simulink model "Time_Varying_Model_2022b"  (R2023b)
settings: Solver=FixedStepAuto  StartTime=0.0  StopTime=10.899  FixedStep=0.01  RelTol=1e-3
values from neighbouring files (symbols this model uses):
  aptos = aptos.calcAeroCoeff(velocity)    [lqr_tuning_analysis.m]    (also in motor_speed_analysis.m; parameter_uncertainty.m; simulator.m; simulator_HIL.m)
  controller = controller.addGain(aptos, steadyState, velocity)    [lqr_tuning_analysis.m]    (also in motor_speed_analysis.m; parameter_uncertainty.m; robustness_analysis.m = controller.addGain(nominal, steadyState, velocity); simulator.m)
  OR = OpenRocketData('openrocket_data/OpenRocket_data_31-03-23.csv')    [robustness_analysis.m]
  q = 0.5 * obj.rho * obj.v^2    [Rocket.m]
  r = aptos    [parameter_uncertainty.m]
undefined symbols (not defined in the file or in its folder): F, Light, MIL
libraries: simulink_extras x20, aerolibutil x1, sharedtransform x1, simulink x1, aerolibwind2 x1
settings Model: Creator=mn19ty  LastModifiedBy=sambr
settings DataIOCC: ReturnWorkspaceOutputsName=yout
settings OptimizationCC: ReuseModelBlockBuffer=off
settings ModelReferenceCC: EnableRefExpFcnMdlSchedulingChecks=on

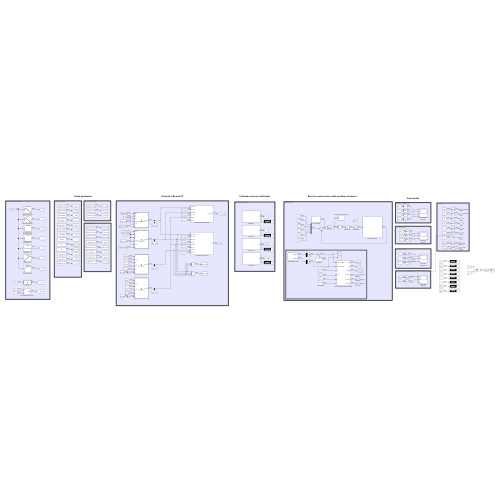
[thumbnail: Simulink's stored preview of the top-level diagram]
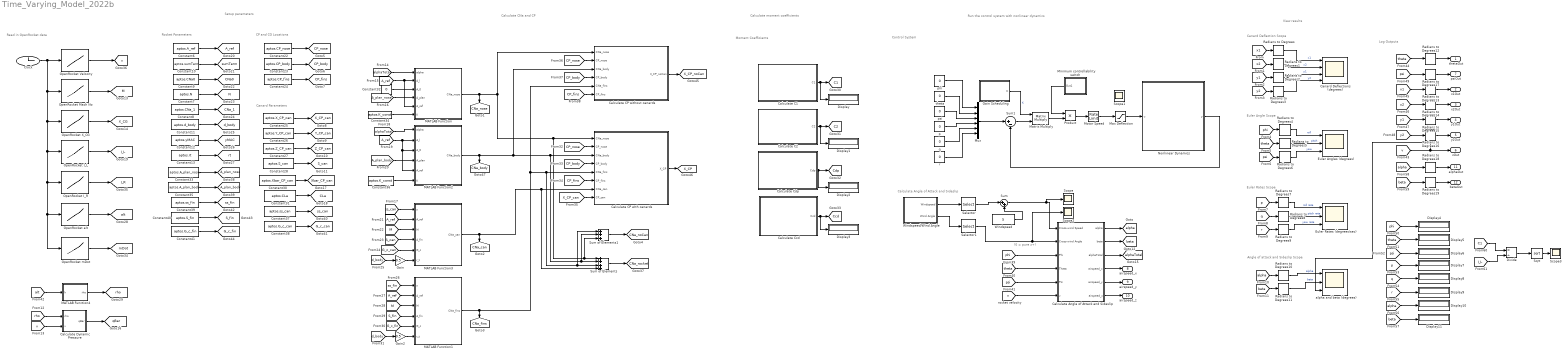
== system Time_Varying_Model_2022b ==
  note: (0 = pure z+)
  note: Log Outputs
  note: Read in OpenRocket data
  note: Calculate Angle of Attack and Sideslip
  note: Angle of attack and Sideslip Scope
  note: View results
  note: Run the control system with nonlinear dynamics
  note: Calculate moment coefficients
  note: Setup parameters
  note: Euler Rates Scope
  note: Euler Angle Scope
  note: Canard Deflection Scope
  note: Control System
  note: Moment Coefficients
  note: Rocket Parameters
  note: Canard Parameters
  note: CP and CG Locations
  note: Calculate CNa and CP
  Calculate Angle of Attack and Sideslip : Subsystem
  Calculate C1 : Subsystem
  Calculate C2 : Subsystem
  Calculate CP with canards : Subsystem
  Calculate CP without canards : Subsystem
  Calculate Ccd : Subsystem
  Calculate Cdp : Subsystem
  Calculate Dynamic Pressure : Subsystem
  Canard Deflections (degrees) : Scope  NumInputPorts=4
  Clock : Clock
  Constant10 : Constant  Value=aptos.sumTerm
  Constant11 : Constant  Value=aptos.d_body
  Constant12 : Constant  Value=aptos.yMAC
  Constant13 : Constant  Value=aptos.rt
  Constant22 : Constant  Value=aptos.CP_nose
  Constant23 : Constant  Value=aptos.CP_body
  Constant24 : Constant  Value=aptos.CP_fins
  Constant25 : Constant  Value=aptos.X_CP_can
  Constant26 : Constant  Value=aptos.Y_CP_can
  Constant27 : Constant  Value=aptos.Z_CP_can
  Constant28 : Constant  Value=aptos.S_can
  Constant30 : Constant  Value=aptos.Xbar_CP_can
  Constant31 : Constant  Value=aptos.CLa
  Constant32 : Constant  Value=0
  Constant33 : Constant  Value=aptos.A_plan_nose
  Constant34 : Constant  Value=aptos.K_const
  Constant35 : Constant  Value=aptos.A_plan_body
  Constant36 : Constant  Value=aptos.K_const
  Constant37 : Constant  Value=aptos.ss_can
  Constant38 : Constant  Value=aptos.G_c_can
  Constant39 : Constant  Value=aptos.ss_fin
  Constant40 : Constant  Value=aptos.S_fin
  Constant41 : Constant  Value=aptos.G_c_fin
  Constant6 : Constant  Value=aptos.A_ref
  Constant7 : Constant  Value=aptos.N
  Constant8 : Constant  Value=aptos.CNa_1
  Constant9 : Constant  Value=aptos.CNa0
  Display{,1..11} (12 alike) : Display
  Divide : Product  Inputs=*/
  Euler Angles (degrees) : Scope  NumInputPorts=3
  Euler Rates (degrees/sec) : Scope  NumInputPorts=3
  Gain : Gain  Gain=0.5
  Gain Scheduling : Subsystem
  Gain2 : Gain  Gain=0.5
  MATLAB Function : MATLAB Function  TreatAsAtomicUnit=on
  MATLAB Function1 : MATLAB Function  TreatAsAtomicUnit=on
  MATLAB Function2 : MATLAB Function  TreatAsAtomicUnit=on
  MATLAB Function3 : MATLAB Function  TreatAsAtomicUnit=on
  MATLAB Function4 : MATLAB Function  TreatAsAtomicUnit=on
  Matrix Multiply : Product  Multiplication=Matrix(*)
  Max Deflection : Saturate  UpperLimit=deg2rad(13)  LowerLimit=-deg2rad(13)
  Minimum controllability switch : Subsystem
  Motor Speed : RateLimiter  RisingSlewLimit=6.54  FallingSlewLimit=-6.54  SampleTimeMode=inherited
  Mux : Mux  Inputs=6
  Nonlinear Dynamics : Subsystem
  OpenRocket I_L : Lookup_n-D  NumberOfTableDimensions=1  BreakpointsForDimension1=OR.t  Table=OR.I_L  InternalRulePriority=Speed  RndMeth=Simplest
  OpenRocket I_R : Lookup_n-D  NumberOfTableDimensions=1  BreakpointsForDimension1=OR.t  Table=OR.I_R  InternalRulePriority=Speed  RndMeth=Simplest
  OpenRocket Mach No : Lookup_n-D  NumberOfTableDimensions=1  BreakpointsForDimension1=OR.t  Table=OR.M  InternalRulePriority=Speed  RndMeth=Simplest
  OpenRocket Velocity : Lookup_n-D  NumberOfTableDimensions=1  BreakpointsForDimension1=OR.t  Table=OR.v  InternalRulePriority=Speed  RndMeth=Simplest
  OpenRocket X_CG : Lookup_n-D  NumberOfTableDimensions=1  BreakpointsForDimension1=OR.t  Table=OR.X_CG  InternalRulePriority=Speed  RndMeth=Simplest
  OpenRocket alt : Lookup_n-D  NumberOfTableDimensions=1  BreakpointsForDimension1=OR.t  Table=OR.h  InternalRulePriority=Speed  RndMeth=Simplest
  OpenRocket mDot : Lookup_n-D  NumberOfTableDimensions=1  BreakpointsForDimension1=OR.t  Table=OR.mDot  InternalRulePriority=Speed  RndMeth=Simplest
  Product : Product
  Radians to Degrees{,1..19} (20 alike) : simulink_extras/Transformations/Radians to Degrees
  Scope{,1..3} (4 alike) : Scope
  Selector : Selector  InputPortWidth=3  IndexOptions=Index vector (dialog)  Indices=[1]  OutputSizes=1
  Selector1 : Selector  InputPortWidth=3  IndexOptions=Index vector (dialog)  Indices=[1]  OutputSizes=1
  Sqrt : Sqrt
  Sum : Sum  Inputs=|++
  Sum of Elements : Sum  Inputs=++++
  Sum of Elements1 : Sum  Inputs=+++
  Sum1 : Sum  Inputs=|+-
  Windspeed : Constant  Value=5
  Windspeed/Wind Angle : Subsystem
  alpha and beta (degrees) : Scope  NumInputPorts=3
  p : Constant  Value=0
  phi : Constant  Value=0
  psi : Constant  Value=0
  q : Constant  Value=0
  r : Constant  Value=0
  theta : Constant  Value=0
  thetaOut : Outport  SignalName=pitchAngle
  x1Out : Outport  Port=2  SignalName=x1
  x2Out : Outport  Port=3  SignalName=x2
  y1Out : Outport  Port=4  SignalName=y1
  y2Out : Outport  Port=5  SignalName=y2
  vOut : Outport  Port=6  SignalName=v
  psiOut : Outport  Port=7  SignalName=yawAngle
  airspeed_x : Outport  Port=8  SignalName=airspeed_x
  airspeed_y : Outport  Port=9  SignalName=airspeed_y
  airspeed_z : Outport  Port=10  SignalName=airspeed_z
  alphaOut : Outport  Port=11  SignalName=alpha
  betaOut : Outport  Port=12  SignalName=beta
  tag scope: A_plan_body=global, A_plan_nose=global, A_ref=global, C1=global, C2=global, CLa=global, CNa0=global, CNa_1=global, CNa_body=global, CNa_can=global, CNa_fins=global, CNa_noCan=global, CNa_nose=global, CNa_rocket=global, CP_body=global, CP_fins=global, CP_nose=global, Ccd=global, Cdp=global, G_c_can=global, G_c_fin=global, I_L=global, I_R=global, M=global, N=global, S_can=global, S_fin=global, X_CG=global, X_CP=global, X_CP_can=global, X_CP_noCan=global, Xbar_CP_can=global, Y_CP_can=global, Z_CP_can=global, alpha=global, alphaTotal=global, alt=global, beta=global, d_body=global, mDot=global, qBar=global, rho=global, rt=global, ss_can=global, ss_fin=global, sumTerm=global, v=global, yMAC=global
  wires:
  Constant22/1 -> [CP_nose]
  Constant23/1 -> [CP_body]
  Constant24/1 -> [CP_fins]
  Constant25/1 -> [X_CP_can]
  Constant26/1 -> [Y_CP_can]
  Constant27/1 -> [Z_CP_can]
  Constant28/1 -> [S_can]
  Constant30/1 -> [Xbar_CP_can]
  Constant31/1 -> [CLa]
  Constant6/1 -> [A_ref]
  Constant10/1 -> [sumTerm]
  Constant9/1 -> [CNa0]
  Constant7/1 -> [N]
  Constant8/1 -> [CNa_1]
  Constant11/1 -> [d_body]
  Constant12/1 -> [yMAC]
  Constant13/1 -> [rt]
  Calculate C1/1(C1) -> Display/1, [C1]
  Calculate C2/1(C2) -> Display1/1, [C2]
  Calculate Cdp/1(Cdp) -> Display2/1, [Cdp]
  Calculate Ccd/1(Ccd) -> Display3/1, [Ccd]
  [x1] -> Radians to Degrees/1
  [y1] -> Radians to Degrees2/1
  [x2] -> Radians to Degrees1/1
  [y2] -> Radians to Degrees3/1
  [theta] -> Radians to Degrees5/1
  [phi] -> Radians to Degrees4/1
  [psi] -> Radians to Degrees6/1
  [q] -> Radians to Degrees8/1
  [p] -> Radians to Degrees7/1
  [r] -> Radians to Degrees9/1
  [alpha] -> Radians to Degrees10/1
  [beta] -> Radians to Degrees11/1
  Sum1/1 -> Matrix Multiply/2
  Nonlinear Dynamics/1(y) -> Sum1/2
  Sum of Elements/1 -> [CNa_rocket]
  MATLAB Function/1(CNa_nose) -> Calculate CP without canards/1(CNa_nose), Calculate CP with canards/1(CNa_nose), Sum of Elements1/3, Sum of Elements/1, [CNa_nose]
  MATLAB Function2/1(CNa_body) -> Sum of Elements1/2, Sum of Elements/2, Calculate CP with canards/3(CNa_body), Calculate CP without canards/3(CNa_body), [CNa_body]
  MATLAB Function3/1(CNa_can) -> [CNa_can], Sum of Elements/4, Calculate CP with canards/7(CNa_can)
  MATLAB Function1/1(CNa_fins) -> [CNa_fins], Calculate CP with canards/5(CNa_fins), Sum of Elements1/1, Sum of Elements/3, Calculate CP without canards/5(CNa_fins)
  Constant32/1 -> MATLAB Function/3(A_0)
  [A_plan_nose] -> MATLAB Function/4(A_plan)
  Constant33/1 -> [A_plan_nose]
  [A_ref] -> MATLAB Function/5(A_ref), MATLAB Function/2(A_l)
  Constant34/1 -> MATLAB Function/6(K)
  [A_ref] -> MATLAB Function2/5(A_ref), MATLAB Function2/3(A_0), MATLAB Function2/2(A_l)
  Constant35/1 -> [A_plan_body]
  [A_plan_body] -> MATLAB Function2/4(A_plan)
  Constant36/1 -> MATLAB Function2/6(K)
  Constant37/1 -> [ss_can]
  [ss_can] -> MATLAB Function3/1(s)
  [A_ref] -> MATLAB Function3/2(A_ref)
  [M] -> MATLAB Function3/3(M)
  [S_can] -> MATLAB Function3/4(A_fin)
  [G_c_can] -> MATLAB Function3/5(G_c)
  Constant38/1 -> [G_c_can]
  [d_body] -> Gain/1
  Gain/1 -> MATLAB Function3/6(r_t)
  Constant39/1 -> [ss_fin]
  [ss_fin] -> MATLAB Function1/1(s)
  [A_ref] -> MATLAB Function1/2(A_ref)
  [M] -> MATLAB Function1/3(M)
  [S_fin] -> MATLAB Function1/4(A_fin)
  Constant40/1 -> [S_fin]
  Constant41/1 -> [G_c_fin]
  [G_c_fin] -> MATLAB Function1/5(G_c)
  Gain2/1 -> MATLAB Function1/6(r_t)
  [d_body] -> Gain2/1
  [CP_nose] -> Calculate CP with canards/2(CP_nose)
  [CP_body] -> Calculate CP with canards/4(CP_body)
  [CP_fins] -> Calculate CP with canards/6(CP_fins)
  [X_CP_can] -> Calculate CP with canards/8(CP_can)
  [CP_nose] -> Calculate CP without canards/2(CP_nose)
  [CP_body] -> Calculate CP without canards/4(CP_body)
  [CP_fins] -> Calculate CP without canards/6(CP_fins)
  Calculate CP without canards/1(X_CP_noCan) -> [X_CP_noCan]
  Calculate CP with canards/1(X_CP) -> [X_CP]
  Sum of Elements1/1 -> [CNa_noCan]
  [alphaTotal] -> MATLAB Function/1(alpha)
  [alphaTotal] -> MATLAB Function2/1(alpha)
  phi/1 -> Mux/1
  theta/1 -> Mux/2
  p/1 -> Mux/4
  q/1 -> Mux/5
  psi/1 -> Mux/3
  r/1 -> Mux/6
  Mux/1 -> Sum1/1
  Windspeed/1 -> Sum/2
  [phi] -> Calculate Angle of Attack and Sideslip/3(Phi)
  [theta] -> Calculate Angle of Attack and Sideslip/4(Theta)
  [psi] -> Calculate Angle of Attack and Sideslip/5(Psi)
  [v] -> Calculate Angle of Attack and Sideslip/6(v)
  Calculate Angle of Attack and Sideslip/1(alpha) -> [alpha]
  Calculate Angle of Attack and Sideslip/2(beta) -> [beta]
  Radians to Degrees/1 -> Canard Deflections (degrees)/1  "x1"
  Radians to Degrees1/1 -> Canard Deflections (degrees)/2  "x2"
  Radians to Degrees2/1 -> Canard Deflections (degrees)/3  "y1"
  Radians to Degrees3/1 -> Canard Deflections (degrees)/4  "y2"
  Radians to Degrees4/1 -> Euler Angles (degrees)/1  "roll"
  Radians to Degrees5/1 -> Euler Angles (degrees)/2  "pitch"
  Radians to Degrees6/1 -> Euler Angles (degrees)/3  "yaw"
  Radians to Degrees7/1 -> Euler Rates (degrees/sec)/1  "roll rate"
  Radians to Degrees8/1 -> Euler Rates (degrees/sec)/2  "pitch rate"
  Radians to Degrees9/1 -> Euler Rates (degrees/sec)/3  "yaw rate"
  Radians to Degrees10/1 -> alpha and beta (degrees)/1  "alpha"
  Radians to Degrees11/1 -> alpha and beta (degrees)/2  "beta"
  OpenRocket Mach No/1 -> [M]
  OpenRocket X_CG/1 -> [X_CG]
  OpenRocket I_L/1 -> [I_L]
  OpenRocket I_R/1 -> [I_R]
  Clock/1 -> OpenRocket Velocity/1, OpenRocket mDot/1, OpenRocket alt/1, OpenRocket I_R/1, OpenRocket I_L/1, OpenRocket X_CG/1, OpenRocket Mach No/1
  [rho] -> Calculate Dynamic Pressure/1(rho)
  [v] -> Calculate Dynamic Pressure/2(v)
  Calculate Dynamic Pressure/1(qBar) -> [qBar]
  OpenRocket alt/1 -> [alt]
  [alt] -> MATLAB Function4/1(h)
  MATLAB Function4/1(rho) -> [rho]
  [theta] -> Radians to Degrees12/1
  Max Deflection/1 -> Nonlinear Dynamics/1(u)
  Motor Speed/1 -> Max Deflection/1
  Radians to Degrees12/1 -> thetaOut/1
  [x1] -> Radians to Degrees13/1
  Radians to Degrees13/1 -> x1Out/1
  [x2] -> Radians to Degrees14/1
  Radians to Degrees14/1 -> x2Out/1
  Radians to Degrees15/1 -> y1Out/1
  [y1] -> Radians to Degrees15/1
  [y2] -> Radians to Degrees16/1
  Radians to Degrees16/1 -> y2Out/1
  Gain Scheduling/1(K) -> Matrix Multiply/1  "K"
  Minimum controllability switch/1(Out1) -> Product/1
  Matrix Multiply/1 -> Product/2
  Product/1 -> Motor Speed/1
  [v] -> alpha and beta (degrees)/3, vOut/1
  Radians to Degrees17/1 -> psiOut/1
  [psi] -> Radians to Degrees17/1
  [phi] -> Display4/1
  [theta] -> Display5/1
  [psi] -> Display6/1
  [p] -> Display7/1
  [q] -> Display8/1
  [r] -> Display9/1
  [alpha] -> Display10/1
  [beta] -> Display11/1
  Calculate Angle of Attack and Sideslip/3(alphaTotal) -> [alphaTotal]
  Calculate Angle of Attack and Sideslip/4(airspeed_x) -> airspeed_x/1
  Calculate Angle of Attack and Sideslip/5(airspeed_y) -> airspeed_y/1
  Calculate Angle of Attack and Sideslip/6(airspeed_z) -> airspeed_z/1
  Radians to Degrees18/1 -> alphaOut/1
  [alpha] -> Radians to Degrees18/1
  [beta] -> Radians to Degrees19/1
  Radians to Degrees19/1 -> betaOut/1
  OpenRocket Velocity/1 -> [v]
  Sum/1 -> Scope/1, Calculate Angle of Attack and Sideslip/1(Cross-wind Speed)
  Windspeed/Wind Angle/1(Windspeed) -> Selector/1
  Selector/1 -> Sum/1
  Windspeed/Wind Angle/2(Wind Angle) -> Selector1/1
  Selector1/1 -> Scope2/1, Calculate Angle of Attack and Sideslip/2(Cross-wind Angle)
  OpenRocket mDot/1 -> [mDot]
  [C1] -> Divide/1
  [I_L] -> Divide/2
  Divide/1 -> Sqrt/1
  Sqrt/1 -> Scope3/1

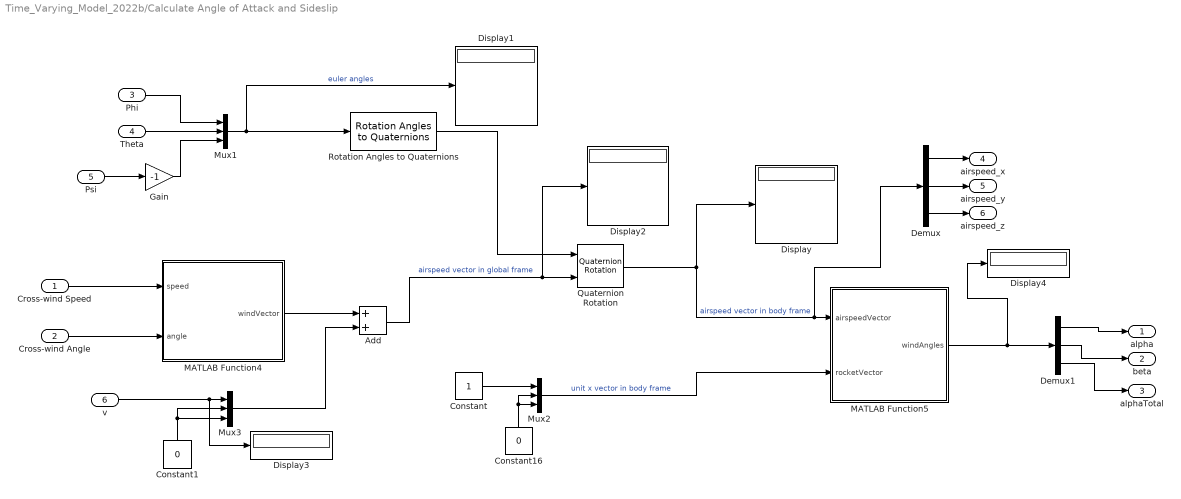
== system Time_Varying_Model_2022b/Calculate Angle of Attack and Sideslip ==
  Cross-wind Speed : Inport
  Cross-wind Angle : Inport  Port=2
  Phi : Inport  Port=3
  Theta : Inport  Port=4
  Psi : Inport  Port=5
  v : Inport  Port=6
  Add : Sum
  Constant : Constant
  Constant1 : Constant  Value=0
  Constant16 : Constant  Value=0
  Demux : Demux  Outputs=3
  Demux1 : Demux  Outputs=3
  Display{,1..4} (5 alike) : Display
  Gain : Gain  Gain=-1
  MATLAB Function4 : MATLAB Function  TreatAsAtomicUnit=on
  MATLAB Function5 : MATLAB Function  TreatAsAtomicUnit=on
  Mux1 : Mux  Inputs=3
  Mux2 : Mux  Inputs=3
  Mux3 : Mux  Inputs=3
  Quaternion Rotation : aerolibutil/Quaternion Rotation
  Rotation Angles to Quaternions : sharedtransform/Rotation Angles to Quaternions  rotationOrder=XYZ  aMode=aMode
  alpha : Outport
  beta : Outport  Port=2
  alphaTotal : Outport  Port=3
  airspeed_x : Outport  Port=4
  airspeed_y : Outport  Port=5
  airspeed_z : Outport  Port=6
  wires:
  Rotation Angles to Quaternions/1 -> Quaternion Rotation/1
  Theta/1 -> Mux1/2
  Mux1/1 -> Rotation Angles to Quaternions/1, Display1/1  "euler angles"
  Phi/1 -> Mux1/1
  Constant16/1 -> Mux2/2, Mux2/3
  MATLAB Function4/1(windVector) -> Add/1
  Demux1/2 -> beta/1
  Cross-wind Angle/1 -> MATLAB Function4/2(angle)
  Cross-wind Speed/1 -> MATLAB Function4/1(speed)
  Psi/1 -> Gain/1
  Constant1/1 -> Mux3/3, Mux3/2
  Mux3/1 -> Add/2
  v/1 -> Display3/1, Mux3/1
  Constant/1 -> Mux2/1
  Demux1/1 -> alpha/1
  MATLAB Function5/1(windAngles) -> Display4/1, Demux1/1
  Add/1 -> Display2/1, Quaternion Rotation/2  "airspeed vector in global frame"
  Quaternion Rotation/1 -> Display/1, Demux/1, MATLAB Function5/1(airspeedVector)  "airspeed vector in body frame"
  Mux2/1 -> MATLAB Function5/2(rocketVector)  "unit x vector in body frame"
  Demux1/3 -> alphaTotal/1
  Demux/1 -> airspeed_x/1
  Demux/2 -> airspeed_y/1
  Demux/3 -> airspeed_z/1
  Gain/1 -> Mux1/3

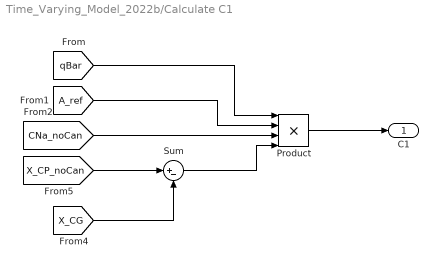
== system Time_Varying_Model_2022b/Calculate C1 ==
  Product : Product  Inputs=4
  Sum : Sum  Inputs=|+-
  C1 : Outport
  wires:
  [X_CP_noCan] -> Sum/1
  [X_CG] -> Sum/2
  Product/1 -> C1/1
  [CNa_noCan] -> Product/3
  [A_ref] -> Product/2
  [qBar] -> Product/1
  Sum/1 -> Product/4

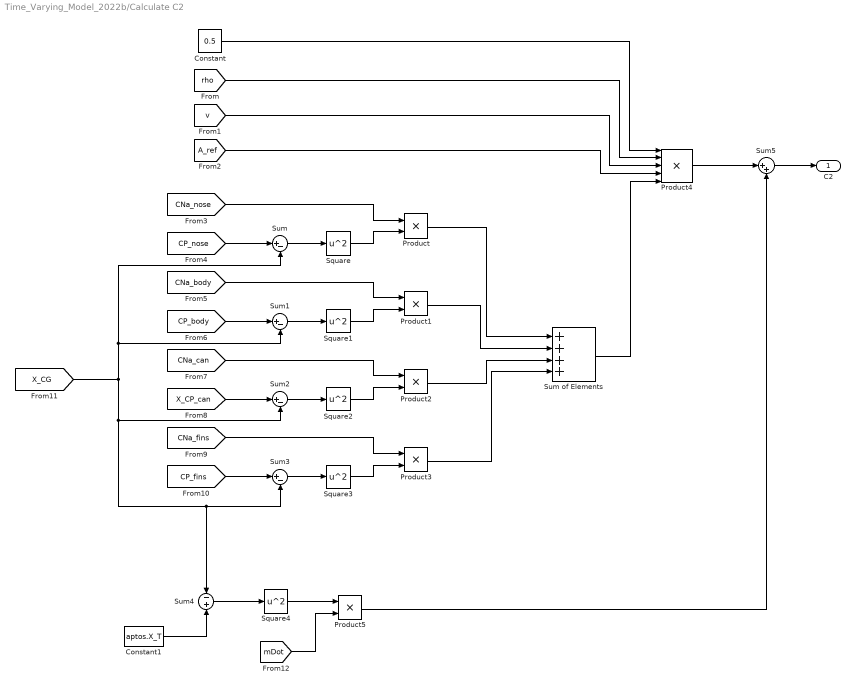
== system Time_Varying_Model_2022b/Calculate C2 ==
  Constant : Constant  Value=0.5
  Constant1 : Constant  Value=aptos.X_T
  Product{,1..3,5} (5 alike) : Product
  Product4 : Product  Inputs=5
  Square{,1..4} (5 alike) : Math  Operator=square
  Sum{,1..3} (4 alike) : Sum  Inputs=|+-
  Sum of Elements : Sum  Inputs=++++
  Sum4 : Sum  Inputs=-+
  Sum5 : Sum  Inputs=|++
  C2 : Outport
  wires:
  [CP_nose] -> Sum/1
  [CP_body] -> Sum1/1
  [X_CP_can] -> Sum2/1
  [CP_fins] -> Sum3/1
  [X_CG] -> Sum4/1, Sum3/2, Sum2/2, Sum/2, Sum1/2
  Sum/1 -> Square/1
  Sum1/1 -> Square1/1
  Sum2/1 -> Square2/1
  Sum3/1 -> Square3/1
  [CNa_nose] -> Product/1
  Square/1 -> Product/2
  Square1/1 -> Product1/2
  [CNa_body] -> Product1/1
  Square2/1 -> Product2/2
  [CNa_can] -> Product2/1
  Square3/1 -> Product3/2
  [CNa_fins] -> Product3/1
  Product/1 -> Sum of Elements/1
  Product1/1 -> Sum of Elements/2
  Product2/1 -> Sum of Elements/3
  Product3/1 -> Sum of Elements/4
  Constant/1 -> Product4/1
  [rho] -> Product4/2
  [v] -> Product4/3
  [A_ref] -> Product4/4
  Sum of Elements/1 -> Product4/5
  Constant1/1 -> Sum4/2
  Sum4/1 -> Square4/1
  Square4/1 -> Product5/1
  [mDot] -> Product5/2
  Product4/1 -> Sum5/1
  Product5/1 -> Sum5/2
  Sum5/1 -> C2/1

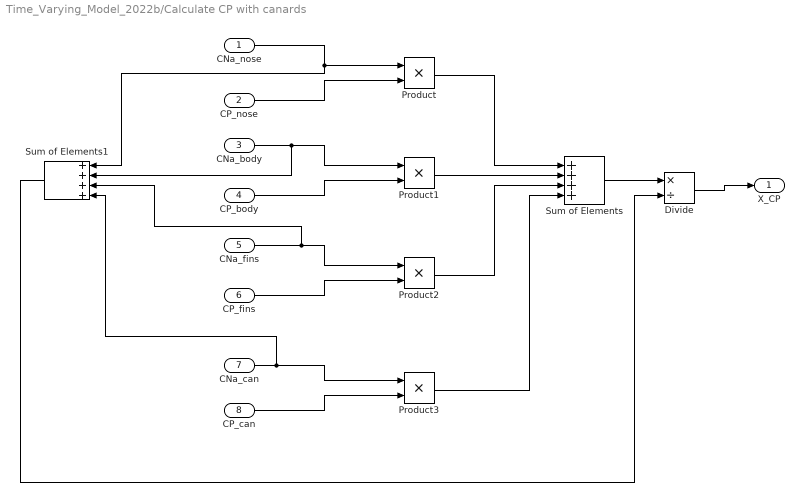
== system Time_Varying_Model_2022b/Calculate CP with canards ==
  CNa_nose : Inport
  CP_nose : Inport  Port=2
  CNa_body : Inport  Port=3
  CP_body : Inport  Port=4
  CNa_fins : Inport  Port=5
  CP_fins : Inport  Port=6
  CNa_can : Inport  Port=7
  CP_can : Inport  Port=8
  Divide : Product  Inputs=*/
  Product{,1..3} (4 alike) : Product
  Sum of Elements : Sum  Inputs=++++
  Sum of Elements1 : Sum  Inputs=++++
  X_CP : Outport
  wires:
  Divide/1 -> X_CP/1
  Sum of Elements1/1 -> Divide/2
  Sum of Elements/1 -> Divide/1
  Product2/1 -> Sum of Elements/3
  Product1/1 -> Sum of Elements/2
  Product/1 -> Sum of Elements/1
  CP_fins/1 -> Product2/2
  CNa_fins/1 -> Sum of Elements1/3, Product2/1
  CP_body/1 -> Product1/2
  CNa_body/1 -> Sum of Elements1/2, Product1/1
  CP_nose/1 -> Product/2
  CNa_nose/1 -> Sum of Elements1/1, Product/1
  CNa_can/1 -> Sum of Elements1/4, Product3/1
  CP_can/1 -> Product3/2
  Product3/1 -> Sum of Elements/4

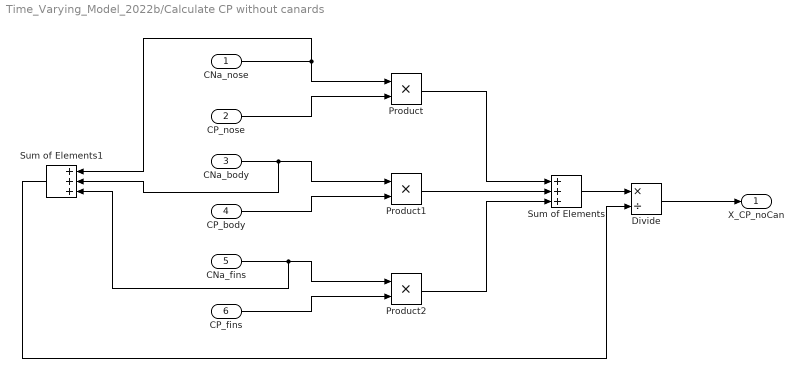
== system Time_Varying_Model_2022b/Calculate CP without canards ==
  CNa_nose : Inport
  CP_nose : Inport  Port=2
  CNa_body : Inport  Port=3
  CP_body : Inport  Port=4
  CNa_fins : Inport  Port=5
  CP_fins : Inport  Port=6
  Divide : Product  Inputs=*/
  Product : Product
  Product1 : Product
  Product2 : Product
  Sum of Elements : Sum  Inputs=+++
  Sum of Elements1 : Sum  Inputs=+++
  X_CP_noCan : Outport
  wires:
  CNa_nose/1 -> Product/1, Sum of Elements1/1
  CP_nose/1 -> Product/2
  CNa_body/1 -> Product1/1, Sum of Elements1/2
  CP_body/1 -> Product1/2
  CNa_fins/1 -> Product2/1, Sum of Elements1/3
  CP_fins/1 -> Product2/2
  Product/1 -> Sum of Elements/1
  Product1/1 -> Sum of Elements/2
  Product2/1 -> Sum of Elements/3
  Sum of Elements/1 -> Divide/1
  Sum of Elements1/1 -> Divide/2
  Divide/1 -> X_CP_noCan/1

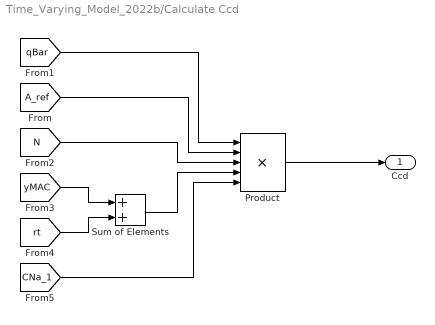
== system Time_Varying_Model_2022b/Calculate Ccd ==
  Product : Product  Inputs=5
  Sum of Elements : Sum
  Ccd : Outport
  wires:
  [yMAC] -> Sum of Elements/1
  [rt] -> Sum of Elements/2
  [qBar] -> Product/1
  [A_ref] -> Product/2
  [N] -> Product/3
  Sum of Elements/1 -> Product/4
  [CNa_1] -> Product/5
  Product/1 -> Ccd/1

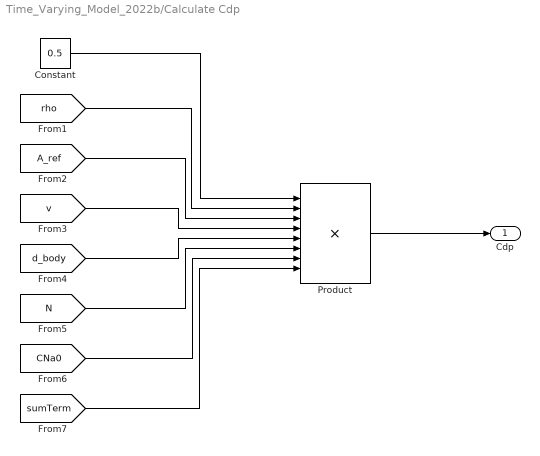
== system Time_Varying_Model_2022b/Calculate Cdp ==
  Constant : Constant  Value=0.5
  Product : Product  Inputs=8
  Cdp : Outport
  wires:
  Product/1 -> Cdp/1
  Constant/1 -> Product/1
  [rho] -> Product/2
  [A_ref] -> Product/3
  [v] -> Product/4
  [d_body] -> Product/5
  [N] -> Product/6
  [CNa0] -> Product/7
  [sumTerm] -> Product/8

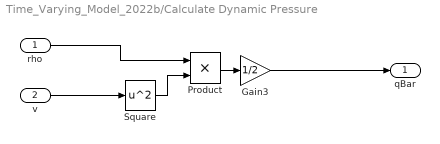
== system Time_Varying_Model_2022b/Calculate Dynamic Pressure ==
  rho : Inport
  v : Inport  Port=2
  Gain3 : Gain  Gain=1/2
  Product : Product
  Square : Math  Operator=square
  qBar : Outport
  wires:
  Product/1 -> Gain3/1
  Gain3/1 -> qBar/1
  Square/1 -> Product/2
  v/1 -> Square/1
  rho/1 -> Product/1

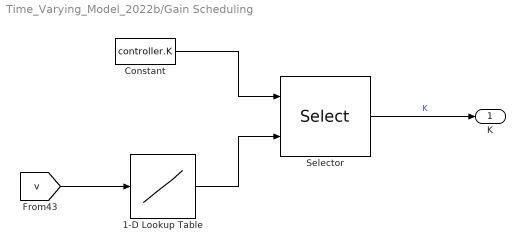
== system Time_Varying_Model_2022b/Gain Scheduling ==
  1-D Lookup Table : Lookup_n-D  NumberOfTableDimensions=1  BreakpointsForDimension1=controller.velocities  Table=1:length(controller.velocities)  InterpMethod=Nearest  InternalRulePriority=Speed  OutDataTypeStr=int8  RndMeth=Simplest
  Constant : Constant  Value=controller.K
  Selector : Selector  NumberOfDimensions=3  InputPortWidth=3  IndexOptions=Select all,Select all,Index vector (port)  Indices=[1 3],1,1  OutputSizes=1,1,1
  K : Outport
  wires:
  [v] -> 1-D Lookup Table/1
  Selector/1 -> K/1  "K"
  1-D Lookup Table/1 -> Selector/2
  Constant/1 -> Selector/1

== system Time_Varying_Model_2022b/Minimum controllability switch ==
  Constant : Constant
  Constant1 : Constant  Value=0
  Switch : Switch  Threshold=controller.minControlSpeed  SaturateOnIntegerOverflow=off  InputSameDT=off
  Out1 : Outport
  wires:
  [v] -> Switch/2
  Switch/1 -> Out1/1
  Constant/1 -> Switch/1
  Constant1/1 -> Switch/3

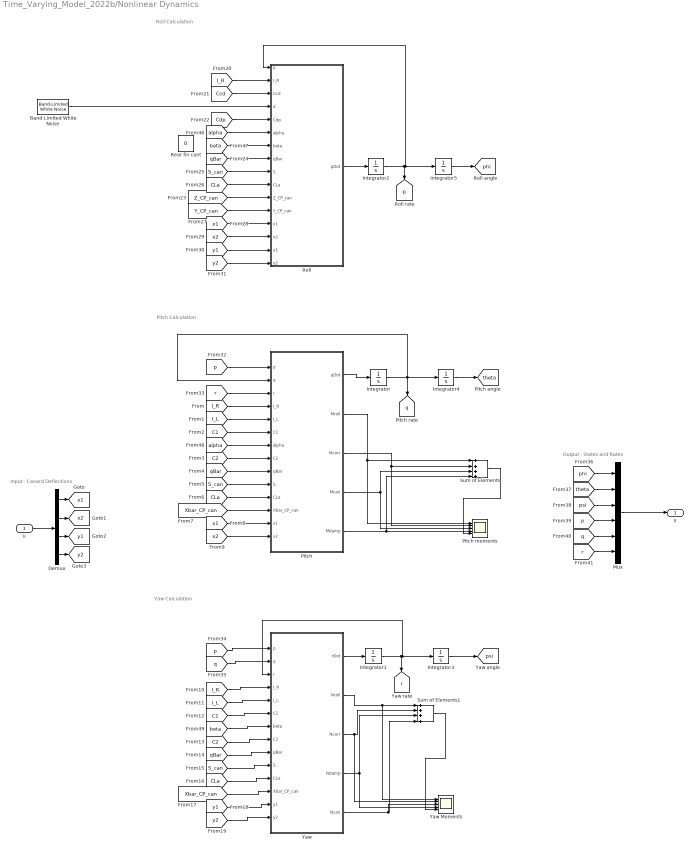
== system Time_Varying_Model_2022b/Nonlinear Dynamics ==
  note: Yaw Calculation
  note: Pitch Calculation
  note: Roll Calculation
  note: Output - States and Rates
  note: Input - Canard Deflections
  u : Inport
  Band-Limited White Noise : simulink/Sources/Band-Limited White Noise  Cov=[0.0001/15]  Ts=0.1  seed=[23341]
  Demux : Demux
  Integrator{,1..5} (6 alike) : Integrator
  Mux : Mux  Inputs=6
  Pitch : MATLAB Function  TreatAsAtomicUnit=on
  Pitch moments : Scope  NumInputPorts=5
  Rear fin cant : Constant  Value=0
  Roll : MATLAB Function  TreatAsAtomicUnit=on
  Sum of Elements : Sum  Inputs=++++
  Sum of Elements1 : Sum  Inputs=++++
  Yaw : MATLAB Function  TreatAsAtomicUnit=on
  Yaw Moments : Scope  NumInputPorts=5
  y : Outport
  tag scope: p=global, phi=global, psi=global, q=global, r=global, theta=global, x1=global, x2=global, y1=global, y2=global
  wires:
  u/1 -> Demux/1
  [I_R] -> Pitch/4(I_R)
  [I_L] -> Pitch/5(I_L)
  [C1] -> Pitch/6(C1)
  [C2] -> Pitch/8(C2)
  [qBar] -> Pitch/9(qBar)
  [S_can] -> Pitch/10(S)
  [CLa] -> Pitch/11(CLa)
  [Xbar_CP_can] -> Pitch/12(Xbar_CP_can)
  Demux/1 -> [x1]
  Demux/2 -> [x2]
  Demux/3 -> [y1]
  Demux/4 -> [y2]
  [x1] -> Pitch/13(x1)
  [x2] -> Pitch/14(x2)
  [y2] -> Yaw/14(y2)
  [y1] -> Yaw/13(y1)
  [Xbar_CP_can] -> Yaw/12(Xbar_CP_can)
  [CLa] -> Yaw/11(CLa)
  [S_can] -> Yaw/10(S)
  [qBar] -> Yaw/9(qBar)
  [C2] -> Yaw/8(C2)
  [C1] -> Yaw/6(C1)
  [I_L] -> Yaw/5(I_L)
  [I_R] -> Yaw/4(I_R)
  Pitch/1(qDot) -> Integrator/1
  Integrator/1 -> Integrator4/1, Pitch/2(q), [q]
  Yaw/1(rDot) -> Integrator1/1
  Integrator1/1 -> Integrator3/1, Yaw/3(r), [r]
  Integrator2/1 -> Roll/1(p), Integrator5/1, [p]
  Roll/1(pDot) -> Integrator2/1
  [x2] -> Roll/14(x2)
  [x1] -> Roll/13(x1)
  [Y_CP_can] -> Roll/12(Y_CP_can)
  [CLa] -> Roll/10(CLa)
  [S_can] -> Roll/9(S)
  [qBar] -> Roll/8(qBar)
  [Z_CP_can] -> Roll/11(Z_CP_can)
  [I_R] -> Roll/2(I_R)
  [Ccd] -> Roll/3(Ccd)
  [Cdp] -> Roll/5(Cdp)
  [y1] -> Roll/15(y1)
  [y2] -> Roll/16(y2)
  [p] -> Pitch/1(p)
  [r] -> Pitch/3(r)
  [p] -> Yaw/1(p)
  [q] -> Yaw/2(q)
  Integrator3/1 -> [psi]
  Integrator4/1 -> [theta]
  Integrator5/1 -> [phi]
  [phi] -> Mux/1
  [theta] -> Mux/2
  [psi] -> Mux/3
  [p] -> Mux/4
  [q] -> Mux/5
  [r] -> Mux/6
  [alpha] -> Roll/6(alpha)
  [beta] -> Roll/7(beta)
  [alpha] -> Pitch/7(alpha)
  [beta] -> Yaw/7(beta)
  Pitch/3(Mcorr) -> Sum of Elements/2, Pitch moments/2
  Pitch/4(Mcan) -> Pitch moments/3, Sum of Elements/3
  Pitch/5(Mdamp) -> Sum of Elements/4, Pitch moments/4
  Sum of Elements/1 -> Pitch moments/5
  Mux/1 -> y/1
  Pitch/2(Mroll) -> Pitch moments/1, Sum of Elements/1
  Yaw/2(Nroll) -> Yaw Moments/1, Sum of Elements1/1
  Yaw/3(Ncorr) -> Yaw Moments/2, Sum of Elements1/2
  Yaw/4(Ndamp) -> Yaw Moments/4, Sum of Elements1/3
  Yaw/5(Ncan) -> Yaw Moments/3, Sum of Elements1/4
  Sum of Elements1/1 -> Yaw Moments/5
  Band-Limited White Noise/1 -> Roll/4(d)

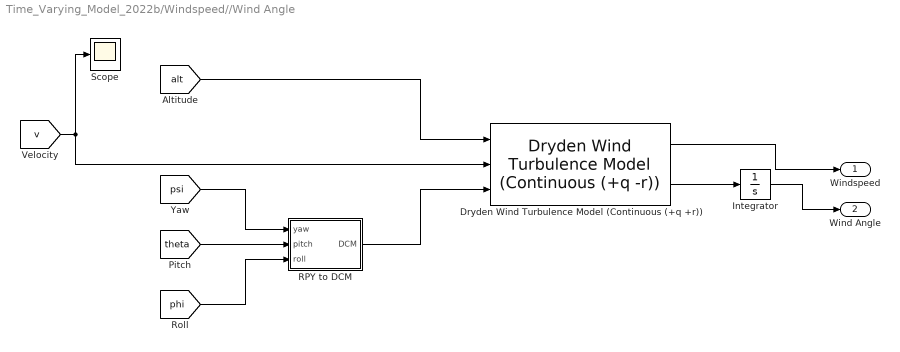
== system Time_Varying_Model_2022b/Windspeed//Wind Angle ==
  Dryden Wind Turbulence Model (Continuous (+q +r)) : aerolibwind2/Dryden Wind Turbulence Model  (Continuous (+q -r))  units=Metric (MKS)  spec=MIL-F-8785C  model=Continuous Dryden (+q +r)  W20=15  Wdeg=0  TurbProb=10^-2 - Light  L_high=533.4  Wingspan=aptos.d_body  ts=0.5  Seed=[23341 23342 23343 23344]  T_on=on
      settings: LibrarySourceBlock=|
      | aerolibwind2/Dryden Wind Turbulence Model
      | (Continuous (+q +r))
  Integrator : Integrator
  RPY to DCM : MATLAB Function  TreatAsAtomicUnit=on
  Scope : Scope
  Windspeed : Outport
  Wind Angle : Outport  Port=2
  wires:
  [psi] -> RPY to DCM/1(yaw)
  [theta] -> RPY to DCM/2(pitch)
  Dryden Wind Turbulence Model (Continuous (+q +r))/1 -> Windspeed/1
  [phi] -> RPY to DCM/3(roll)
  [alt] -> Dryden Wind Turbulence Model (Continuous (+q +r))/1
  RPY to DCM/1(DCM) -> Dryden Wind Turbulence Model (Continuous (+q +r))/3
  [v] -> Scope/1, Dryden Wind Turbulence Model (Continuous (+q +r))/2
  Dryden Wind Turbulence Model (Continuous (+q +r))/2 -> Integrator/1
  Integrator/1 -> Wind Angle/1

== matlab function Time_Varying_Model_2022b/MATLAB Function1 ==
  data: s input; A_ref input; CNa_fins output; M input; A_fin input; G_c input; r_t input
% CNa for fins
function CNa_fins = findCNaFins(s, A_ref, M, A_fin, G_c, r_t)

    CNa1_num = 2*pi()*(s^2/A_ref);                                       %numerator
    CNa1_den = 1 + sqrt(1+(((s^2)*sqrt(1-M^2))/(A_fin*cos(G_c)))^2);     %denominator
    
    CNa1 = CNa1_num / CNa1_den;    %one fin

    CNa4 = 2*CNa1;                 %all fins
    
    K_TB = 1 + r_t/(s+r_t);        %interference correction factor
    
    CNa_fins = K_TB*CNa4; 
    
end

== matlab function Time_Varying_Model_2022b/MATLAB Function2 ==
  data: alpha input; CNa_body output; A_l input; A_0 input; A_plan input; A_ref input; K input
% CNa for body components
function CNa_body = findCNaBody(alpha, A_l, A_0, A_plan, A_ref, K)
    
    %Apply limit conditions
    if alpha == 0
        
        a1 = 1;
        a2 = 0;
        
    else 
       
        a1  = sin(alpha)/alpha;
        a2  = (sin(alpha)^2)/alpha;
        
    end
    
    CNa_body = (2/A_ref)*(A_l-A_0)*a1+K*(A_plan/A_ref)*a2;

end

== matlab function Time_Varying_Model_2022b/MATLAB Function3 ==
  data: s input; A_ref input; CNa_can output; M input; A_fin input; G_c input; r_t input
% CNa for fins
function CNa_can = findCNaCan(s, A_ref, M, A_fin, G_c, r_t)

    CNa1_num = 2*pi()*(s^2/A_ref);                                       %numerator
    CNa1_den = 1 + sqrt(1+(((s^2)*sqrt(1-M^2))/(A_fin*cos(G_c)))^2);     %denominator
    
    CNa1 = CNa1_num / CNa1_den;    %one fin

    CNa4 = 2*CNa1;                 %all fins
    
    K_TB = 1 + r_t/(s+r_t);        %interference correction factor
    
    CNa_can = K_TB*CNa4; 
    
end

== matlab function Time_Varying_Model_2022b/Calculate Angle of Attack and Sideslip/MATLAB Function4 ==
  data: speed input size=[1 1]; windVector output size=[3 1]; angle input size=[1 1]
function windVector = findWindVector(speed, angle)

ang_cos = cos(angle);
ang_sin = sin(angle);

if abs(ang_cos) < 1e-4
    ang_cos = 0;
end

if abs(ang_sin) < 1e-4
    ang_sin = 0;
end

windVector = [0; speed*ang_sin; speed*ang_cos];

== matlab function Time_Varying_Model_2022b/Calculate Angle of Attack and Sideslip/MATLAB Function5 ==
  data: airspeedVector input double size=[3 1]; windAngles output double size=[3 1]; rocketVector input double size=[3 1]
function windAngles = findWindAngles(airspeedVector, rocketVector)
    
    % Find projections in xy and xz planes
    airspeedVector_xy = [airspeedVector(1); airspeedVector(2); 0];
    airspeedVector_xz = [airspeedVector(1); 0; airspeedVector(3)];

    alpha = atan2(airspeedVector_xz(3), airspeedVector_xz(1));
    beta = atan2(airspeedVector_xy(2), airspeedVector_xy(1));

    alphaTotal = acos(dot(airspeedVector, rocketVector)/(norm(airspeedVector)*norm(rocketVector)));

%     alpha = acos(dot(airspeedVector_xz, rocketVector)/(norm(airspeedVector_xz)*norm(rocketVector)));
%     beta = acos(dot(airspeedVector_xy, rocketVector)/(norm(airspeedVector_xy)*norm(rocketVector)));

% angles = [aboutZ, aboutY, aboutX]
windAngles = [alpha; beta; alphaTotal];      % = [alpha; beta]

== matlab function Time_Varying_Model_2022b/MATLAB Function4 ==
  data: h input; rho output
function rho = calcRho(h)     % Calculate air density using ISA values

    % Define constants
    T0 = 288.15;    % SL temp (K)
    rho0 = 1.2256;  % SL density (kg/m3)
    L = 0.0065;     % Lapse rate (K/m)
    g = 9.81;
    R = 287.26;     % Gas constant (J/kg/K)
    
rho = rho0*((T0-L*h)/T0)^((g/(L*R))-1);

== matlab function Time_Varying_Model_2022b/Windspeed//Wind Angle/RPY to DCM ==
  data: yaw input; pitch input; roll input; DCM output
function DCM = fcn(yaw, pitch, roll)

coder.extrinsic('angle2dcm');

DCM=zeros(3);

DCM = angle2dcm(yaw,pitch,roll);

== matlab function Time_Varying_Model_2022b/Nonlinear Dynamics/Yaw ==
  data: p input; q input; r input; I_R input; rDot output; I_L input; C1 input; beta input; C2 input; qBar input; S input; CLa input; Xbar_CP_can input; y1 input; y2 input; Nroll output; Ncorr output; Ndamp output; Ncan output
function [rDot, Nroll, Ncorr, Ndamp, Ncan] = calcrDot(p, q, r, I_R, I_L, C1, beta, C2, qBar, S, CLa, Xbar_CP_can, y1, y2)

Nroll = -((I_L-I_R)/I_L)*p*q;

Ncorr = -(C1/I_L)*beta;

Ndamp = -(C2/I_L)*r;

Ncan = ((qBar*S*CLa*Xbar_CP_can)/I_L)*((beta+y1)*cos(y1)+(beta-y2)*cos(y2));

rDot = Nroll + Ncorr + Ndamp + Ncan;

== matlab function Time_Varying_Model_2022b/Nonlinear Dynamics/Pitch ==
  data: p input; q input; r input; I_R input; qDot output; Mroll output; I_L input; C1 input; alpha input; C2 input; qBar input; S input; CLa input; Xbar_CP_can input; x1 input; x2 input; Mcorr output; Mcan output; Mdamp output
function [qDot, Mroll, Mcorr, Mcan, Mdamp] = calcqDot(p, q, r, I_R, I_L, C1, alpha, C2, qBar, S, CLa, Xbar_CP_can, x1, x2)

Mroll = -((I_R-I_L)/I_L)*p*r;

Mcorr = -(C1/I_L)*alpha;

Mcan = ((qBar*S*CLa*Xbar_CP_can)/I_L)*((alpha+x1)*cos(x1)+(alpha-x2)*cos(x2));

Mdamp = -(C2/I_L)*q;

qDot = Mroll + Mcorr + Mcan + Mdamp;

== matlab function Time_Varying_Model_2022b/Nonlinear Dynamics/Roll ==
  data: p input; I_R input; Ccd input; d input; pDot output; Cdp input; alpha input; beta input; qBar input; S input; CLa input; Z_CP_can input; Y_CP_can input; x1 input; x2 input; y1 input; y2 input
function pDot = calcpDot(p, I_R, Ccd, d, Cdp, alpha, beta, qBar, S, CLa, Z_CP_can, Y_CP_can, x1, x2, y1, y2)

pDot = (Ccd/I_R)*d - (Cdp/I_R)*p + ((qBar*S*CLa)/I_R)*(Z_CP_can*((alpha+x1)*cos(x1)+(x2-alpha)*cos(x2))+Y_CP_can*((beta+y1)*cos(y1)+(y2-beta)*cos(y2)));

== matlab function Time_Varying_Model_2022b/MATLAB Function ==
  data: alpha input; CNa_nose output; A_l input; A_0 input; A_plan input; A_ref input; K input
% CNa for body components
function CNa_nose = findCNaNose(alpha, A_l, A_0, A_plan, A_ref, K)
    
    %Apply limit conditions
    if alpha == 0
        
        a1 = 1;
        a2 = 0;
        
    else 
       
        a1  = sin(alpha)/alpha;
        a2  = (sin(alpha)^2)/alpha;
        
    end
    
    CNa_nose = (2/A_ref)*(A_l-A_0)*a1+K*(A_plan/A_ref)*a2;

end
